simulink model "twip_control"  (R2015a)
settings: Solver=ode45  StartTime=0.0  StopTime=10  RelTol=1e-3
values from neighbouring files (symbols this model uses):
  s1 = 0.15    [Fuzzy_Balance_Controller_Mamdani.m]    (also in twip_sys.m = 1)
  s1_y = 0.5    [Fuzzy_Yaw_Controller_Mamdani.m]
  s2 = 0.4    [Fuzzy_Balance_Controller_Mamdani.m]    (also in twip_sys.m = 1)
  s2_y = 0.5    [Fuzzy_Yaw_Controller_Mamdani.m]
libraries: simulink x3, fuzblock x2
settings Model: Creator=elew  LastModifiedBy=ignacio
settings OptimizationCC: BlockReduction=off  OptimizeBlockIOStorage=off  BufferReuse=off  GlobalBufferReuse=off  ExpressionFolding=off  LocalBlockOutputs=off

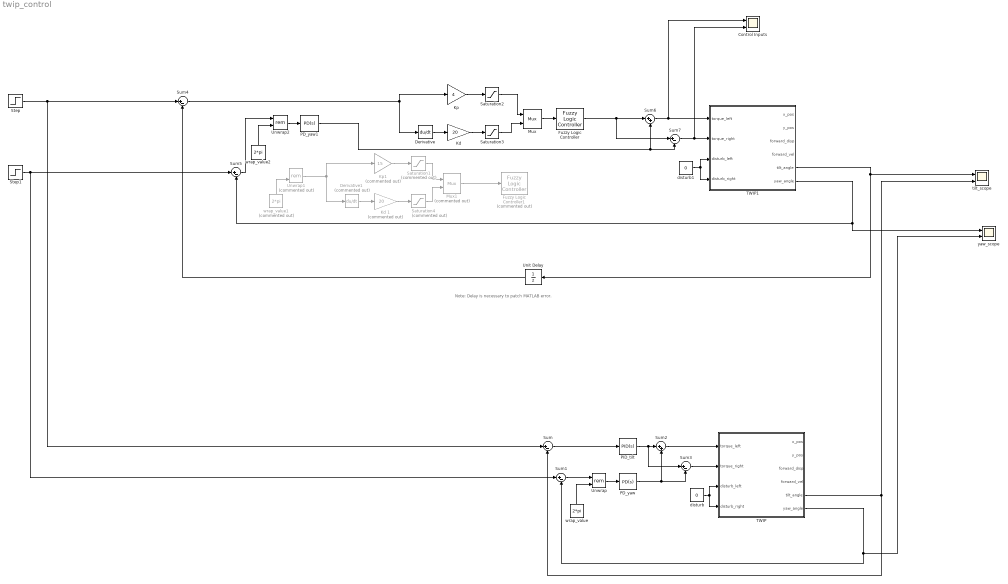
== system twip_control ==
  note: Note: Delay is necessary to patch MATLAB error.
  Control Inputs : Scope  NumInputPorts=2
      settings: YMin=-2~-2  YMax=1.5~1.5  SaveName=ScopeData2
  Derivative : Derivative
  Derivative1 : Derivative  Commented=on
  Fuzzy Logic Controller : fuzblock/Fuzzy Logic  Controller  fis='Bal.fis'
  Fuzzy Logic Controller1 : fuzblock/Fuzzy Logic  Controller  Commented=on  fis='Yaw.fis'
  "Kd " : Gain  Gain=20
  Kd 1 : Gain  Commented=on  Gain=20
  Kp : Gain  Gain=4
  Kp1 : Gain  Commented=on  Gain=15
  Mux : Mux  Inputs=2
      settings: DisplayOption=signals
  Mux1 : Mux  Commented=on  Inputs=2
      settings: DisplayOption=signals
  PD_yaw : simulink/Continuous/PID Controller  Controller=PD  TimeDomain=Continuous-time  SampleTime=-1  IntegratorMethod=Forward Euler  FilterMethod=Forward Euler  Form=Parallel  UseFilter=on  ControllerParametersSource=internal  P=25  I=100  D=1  N=100  InitialConditionSource=internal  InitialConditionForIntegrator=0  InitialConditionForFilter=0  ExternalReset=none  LimitOutput=off  UpperSaturationLimit=inf  LowerSaturationLimit=-inf  LinearizeAsGain=on  AntiWindupMode=none  Kb=1  TrackingMode=off  Kt=1  PParamMin=[]  PParamMax=[]  IParamMin=[]  IParamMax=[]  DParamMin=[]  DParamMax=[]  NParamMin=[]  NParamMax=[]  KbParamMin=[]  KbParamMax=[]  KtParamMin=[]  KtParamMax=[]  POutMin=[]  POutMax=[]  IOutMin=[]  IOutMax=[]  DOutMin=[]  DOutMax=[]  NOutMin=[]  NOutMax=[]  KbOutMin=[]  KbOutMax=[]  KtOutMin=[]  KtOutMax=[]  IntegratorOutMin=[]  IntegratorOutMax=[]  FilterOutMin=[]  FilterOutMax=[]  SumOutMin=[]  SumOutMax=[]  SumI1OutMin=[]  SumI1OutMax=[]  SumI2OutMin=[]  SumI2OutMax=[]  SumI3OutMin=[]  SumI3OutMax=[]  SumDOutMin=[]  SumDOutMax=[]  SaturationOutMin=[]  SaturationOutMax=[]  IntegratorContinuousStateAttributes=''  IntegratorStateMustResolveToSignalObject=off  IntegratorRTWStateStorageClass=Auto  FilterContinuousStateAttributes=''  FilterStateMustResolveToSignalObject=off  FilterRTWStateStorageClass=Auto  DifferentiatorICPrevScaledInput=0  DifferentiatorOutMin=[]  DifferentiatorOutMax=[]
  PD_yaw1 : simulink/Continuous/PID Controller  Controller=PD  TimeDomain=Continuous-time  SampleTime=-1  IntegratorMethod=Forward Euler  FilterMethod=Forward Euler  Form=Parallel  UseFilter=on  ControllerParametersSource=internal  P=25  I=100  D=1  N=100  InitialConditionSource=internal  InitialConditionForIntegrator=0  InitialConditionForFilter=0  ExternalReset=none  LimitOutput=off  UpperSaturationLimit=inf  LowerSaturationLimit=-inf  LinearizeAsGain=on  AntiWindupMode=none  Kb=1  TrackingMode=off  Kt=1  PParamMin=[]  PParamMax=[]  IParamMin=[]  IParamMax=[]  DParamMin=[]  DParamMax=[]  NParamMin=[]  NParamMax=[]  KbParamMin=[]  KbParamMax=[]  KtParamMin=[]  KtParamMax=[]  POutMin=[]  POutMax=[]  IOutMin=[]  IOutMax=[]  DOutMin=[]  DOutMax=[]  NOutMin=[]  NOutMax=[]  KbOutMin=[]  KbOutMax=[]  KtOutMin=[]  KtOutMax=[]  IntegratorOutMin=[]  IntegratorOutMax=[]  FilterOutMin=[]  FilterOutMax=[]  SumOutMin=[]  SumOutMax=[]  SumI1OutMin=[]  SumI1OutMax=[]  SumI2OutMin=[]  SumI2OutMax=[]  SumI3OutMin=[]  SumI3OutMax=[]  SumDOutMin=[]  SumDOutMax=[]  SaturationOutMin=[]  SaturationOutMax=[]  IntegratorContinuousStateAttributes=''  IntegratorStateMustResolveToSignalObject=off  IntegratorRTWStateStorageClass=Auto  FilterContinuousStateAttributes=''  FilterStateMustResolveToSignalObject=off  FilterRTWStateStorageClass=Auto  DifferentiatorICPrevScaledInput=0  DifferentiatorOutMin=[]  DifferentiatorOutMax=[]
  PID_tilt : simulink/Continuous/PID Controller  Controller=PID  TimeDomain=Continuous-time  SampleTime=-1  IntegratorMethod=Forward Euler  FilterMethod=Forward Euler  Form=Parallel  UseFilter=on  ControllerParametersSource=internal  P=50  I=100  D=2  N=100  InitialConditionSource=internal  InitialConditionForIntegrator=0  InitialConditionForFilter=0  ExternalReset=none  LimitOutput=off  UpperSaturationLimit=inf  LowerSaturationLimit=-inf  LinearizeAsGain=on  AntiWindupMode=none  Kb=1  TrackingMode=off  Kt=1  PParamMin=[]  PParamMax=[]  IParamMin=[]  IParamMax=[]  DParamMin=[]  DParamMax=[]  NParamMin=[]  NParamMax=[]  KbParamMin=[]  KbParamMax=[]  KtParamMin=[]  KtParamMax=[]  POutMin=[]  POutMax=[]  IOutMin=[]  IOutMax=[]  DOutMin=[]  DOutMax=[]  NOutMin=[]  NOutMax=[]  KbOutMin=[]  KbOutMax=[]  KtOutMin=[]  KtOutMax=[]  IntegratorOutMin=[]  IntegratorOutMax=[]  FilterOutMin=[]  FilterOutMax=[]  SumOutMin=[]  SumOutMax=[]  SumI1OutMin=[]  SumI1OutMax=[]  SumI2OutMin=[]  SumI2OutMax=[]  SumI3OutMin=[]  SumI3OutMax=[]  SumDOutMin=[]  SumDOutMax=[]  SaturationOutMin=[]  SaturationOutMax=[]  IntegratorContinuousStateAttributes=''  IntegratorStateMustResolveToSignalObject=off  IntegratorRTWStateStorageClass=Auto  FilterContinuousStateAttributes=''  FilterStateMustResolveToSignalObject=off  FilterRTWStateStorageClass=Auto  DifferentiatorICPrevScaledInput=0  DifferentiatorOutMin=[]  DifferentiatorOutMax=[]
  Saturation1 : Saturate  Commented=on  UpperLimit=1*s1_y  LowerLimit=-1*s1_y  ZeroCross=off
  Saturation2 : Saturate  UpperLimit=6*s1  LowerLimit=-6*s1  ZeroCross=off
  Saturation3 : Saturate  UpperLimit=2*s2  LowerLimit=-2*s2  ZeroCross=off
  Saturation4 : Saturate  Commented=on  UpperLimit=1*s2_y  LowerLimit=-1*s2_y  ZeroCross=off
  Step : Step  After=-0.3  SampleTime=0
  Step1 : Step  After=0.1  SampleTime=0
  Sum{,1,3..5,7} (6 alike) : Sum  Inputs=|+-
  Sum2 : Sum  Inputs=|++
  Sum6 : Sum  Inputs=|++
  TWIP : Subsystem
      mask Display:
      | image('twip_mask.png')
      | port_label('input', 1, 'torque_l')
      | port_label('input', 2, 'torque_r')
      | port_label('input', 3, 'disturb_l')
      | port_label('input', 4, 'disturb_r')
      | 
      | 
      | port_label('output', 1, 'x_pos')
      | port_label('output', 2, 'y_pos')
      | port_label('output', 3, 'disp')
      | port_label('output', 4, 'vel')
      | port_label('output', 5, 'tilt')
      | port_label('output', 6, 'yaw')
  TWIP1 : Subsystem
      mask Display:
      | image('twip_mask.png')
      | port_label('input', 1, 'torque_l')
      | port_label('input', 2, 'torque_r')
      | port_label('input', 3, 'disturb_l')
      | port_label('input', 4, 'disturb_r')
      | 
      | 
      | port_label('output', 1, 'x_pos')
      | port_label('output', 2, 'y_pos')
      | port_label('output', 3, 'disp')
      | port_label('output', 4, 'vel')
      | port_label('output', 5, 'tilt')
      | port_label('output', 6, 'yaw')
  Unit Delay : UnitDelay  SampleTime=0.01
  Unwrap : Math  Operator=rem  SaturateOnIntegerOverflow=on
  Unwrap1 : Math  Commented=on  Operator=rem  SaturateOnIntegerOverflow=on
  Unwrap2 : Math  Operator=rem  SaturateOnIntegerOverflow=on
  disturb : Constant  Value=0
  disturb1 : Constant  Value=0
  "tilt_scope " : Scope  NumInputPorts=2
      settings: ShowLegends=on  TimeRange=2.2890625  YMin=-0.303~-0.301  YMax=-0.29775~-0.2915  SaveName=ScopeData4
  wrap_value : Constant  Value=2*pi
  wrap_value1 : Constant  Commented=on  Value=2*pi
  wrap_value2 : Constant  Value=2*pi
  yaw_scope : Scope  NumInputPorts=2
      settings: YMin=0.1~0.1  YMax=0.1~0.1  SaveName=ScopeData5
  wires:
  TWIP/5(tilt_angle) -> Sum/2, "tilt_scope "/2
  Sum/1 -> PID_tilt/1
  disturb/1 -> TWIP/4(disturb_right), TWIP/3(disturb_left)
  TWIP/6(yaw_angle) -> yaw_scope/2, Sum1/2
  Sum1/1 -> Unwrap/1
  Sum2/1 -> TWIP/1(torque_left)
  Sum3/1 -> TWIP/2(torque_right)
  Unwrap/1 -> PD_yaw/1
  wrap_value/1 -> Unwrap/2
  disturb1/1 -> TWIP1/4(disturb_right), TWIP1/3(disturb_left)
  Sum7/1 -> Control Inputs/2, TWIP1/2(torque_right)
  wrap_value1/1 -> Unwrap1/2
  TWIP1/5(tilt_angle) -> Unit Delay/1, "tilt_scope "/1
  Derivative/1 -> "Kd "/1
  Unit Delay/1 -> Sum4/2
  Sum4/1 -> Derivative/1, Kp/1
  Mux/1 -> Fuzzy Logic Controller/1
  Kp/1 -> Saturation2/1
  "Kd "/1 -> Saturation3/1
  Saturation2/1 -> Mux/1
  Saturation3/1 -> Mux/2
  Derivative1/1 -> Kd 1/1
  Unwrap1/1 -> Kp1/1, Derivative1/1
  Mux1/1 -> Fuzzy Logic Controller1/1
  Kp1/1 -> Saturation1/1
  Kd 1/1 -> Saturation4/1
  Saturation1/1 -> Mux1/1
  Saturation4/1 -> Mux1/2
  PID_tilt/1 -> Sum3/1, Sum2/1
  Step/1 -> Sum/1, Sum4/1
  Step1/1 -> Sum5/1, Sum1/1
  Sum5/1 -> Unwrap2/1
  Unwrap2/1 -> PD_yaw1/1
  wrap_value2/1 -> Unwrap2/2
  Fuzzy Logic Controller/1 -> Sum7/1, Sum6/1
  PD_yaw/1 -> Sum3/2, Sum2/2
  Sum6/1 -> Control Inputs/1, TWIP1/1(torque_left)
  PD_yaw1/1 -> Sum7/2, Sum6/2
  TWIP1/6(yaw_angle) -> Sum5/2, yaw_scope/1

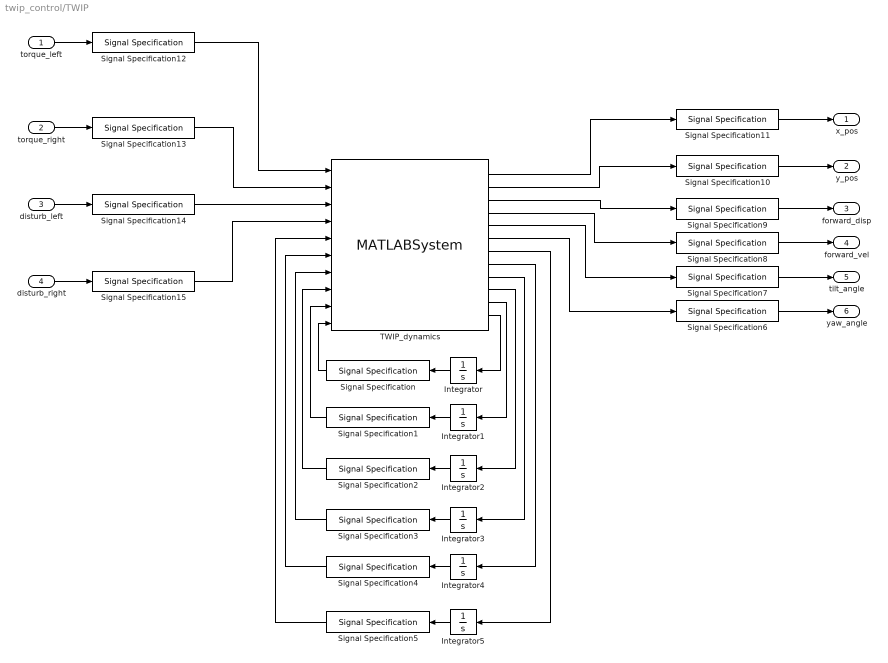
== system twip_control/TWIP ==
  torque_left : Inport
  torque_right : Inport  Port=2
  disturb_left : Inport  Port=3
  disturb_right : Inport  Port=4
  Integrator{,1..4} (5 alike) : Integrator
  Integrator5 : Integrator  InitialCondition=0.3
  Signal Specification{,1..15} (16 alike) : SignalSpecification  Dimensions=[1]
  TWIP_dynamics : MATLABSystem  System=twip_sys  M=[0.5]  Mw=[0.8]  mm=[0.5]  Iw=[0.02]  Ip=[0.06]  Imm=[0.08]  r=[0.2]  l=[0.15]  d=[0.6]  SimulateUsing=Interpreted execution
      mask Type: twip_sys
      mask Display:
      | disp('twip_sys');
      | port_label('input',1,'tl');
      | port_label('input',2,'tr');
      | port_label('input',3,'dl');
      | port_label('input',4,'dr');
      | port_label('input',5,'y1');
      | port_label('input',6,'y2');
      | port_label('input',7,'y3');
      | port_label('input',8,'y4');
      | port_label('input',9,'y5');
      | port_label('input',10,'y6');
      | port_label('output',1,'x');
      | port_label('output',2,'y');
      | port_label('output',3,'xp');
      | port_label('output',4,'v');
      | port_label('output',5,'alpha');
      | port_label('output',6,'theta');
      | port_label('output',7,'yd1');
      | port_label('output',8,'yd2');
      | port_label('output',9,'yd3');
      | port_label('output',10,'yd4');
      | port_label('output',11,'yd5');
      | port_label('output',12,'yd6');
  x_pos : Outport
  y_pos : Outport  Port=2
  forward_disp : Outport  Port=3
  forward_vel : Outport  Port=4
  tilt_angle : Outport  Port=5
  yaw_angle : Outport  Port=6
  wires:
  torque_right/1 -> Signal Specification13/1
  torque_left/1 -> Signal Specification12/1
  disturb_right/1 -> Signal Specification15/1
  disturb_left/1 -> Signal Specification14/1
  TWIP_dynamics/1 -> Signal Specification11/1
  TWIP_dynamics/2 -> Signal Specification10/1
  TWIP_dynamics/3 -> Signal Specification9/1
  TWIP_dynamics/4 -> Signal Specification8/1
  TWIP_dynamics/5 -> Signal Specification7/1
  TWIP_dynamics/6 -> Signal Specification6/1
  TWIP_dynamics/12 -> Integrator/1
  Integrator/1 -> Signal Specification/1
  Integrator1/1 -> Signal Specification1/1
  Integrator2/1 -> Signal Specification2/1
  Integrator3/1 -> Signal Specification3/1
  Integrator4/1 -> Signal Specification4/1
  Integrator5/1 -> Signal Specification5/1
  TWIP_dynamics/11 -> Integrator1/1
  TWIP_dynamics/10 -> Integrator2/1
  TWIP_dynamics/9 -> Integrator3/1
  TWIP_dynamics/8 -> Integrator4/1
  TWIP_dynamics/7 -> Integrator5/1
  Signal Specification/1 -> TWIP_dynamics/10
  Signal Specification1/1 -> TWIP_dynamics/9
  Signal Specification2/1 -> TWIP_dynamics/8
  Signal Specification3/1 -> TWIP_dynamics/7
  Signal Specification4/1 -> TWIP_dynamics/6
  Signal Specification5/1 -> TWIP_dynamics/5
  Signal Specification6/1 -> yaw_angle/1
  Signal Specification7/1 -> tilt_angle/1
  Signal Specification8/1 -> forward_vel/1
  Signal Specification9/1 -> forward_disp/1
  Signal Specification10/1 -> y_pos/1
  Signal Specification11/1 -> x_pos/1
  Signal Specification12/1 -> TWIP_dynamics/1
  Signal Specification13/1 -> TWIP_dynamics/2
  Signal Specification14/1 -> TWIP_dynamics/3
  Signal Specification15/1 -> TWIP_dynamics/4

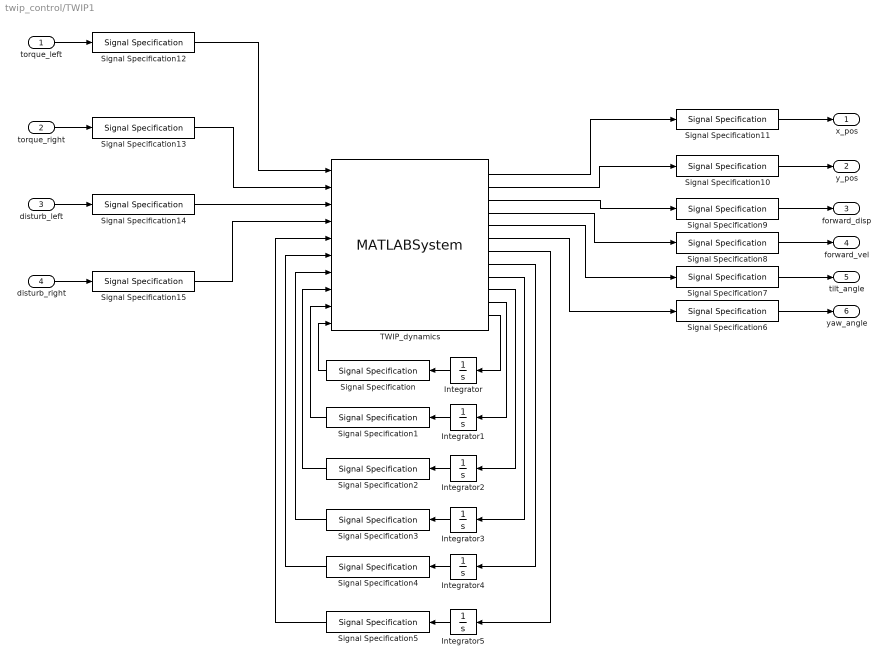
== system twip_control/TWIP1 ==
  torque_left : Inport
  torque_right : Inport  Port=2
  disturb_left : Inport  Port=3
  disturb_right : Inport  Port=4
  Integrator{,1..4} (5 alike) : Integrator
  Integrator5 : Integrator  InitialCondition=0.3
  Signal Specification{,1..15} (16 alike) : SignalSpecification  Dimensions=[1]
  TWIP_dynamics : MATLABSystem  System=twip_sys  M=[0.5]  Mw=[0.8]  mm=[0.5]  Iw=[0.02]  Ip=[0.06]  Imm=[0.08]  r=[0.2]  l=[0.15]  d=[0.6]  SimulateUsing=Interpreted execution
      mask Type: twip_sys
      mask Display:
      | disp('twip_sys');
      | port_label('input',1,'tl');
      | port_label('input',2,'tr');
      | port_label('input',3,'dl');
      | port_label('input',4,'dr');
      | port_label('input',5,'y1');
      | port_label('input',6,'y2');
      | port_label('input',7,'y3');
      | port_label('input',8,'y4');
      | port_label('input',9,'y5');
      | port_label('input',10,'y6');
      | port_label('output',1,'x');
      | port_label('output',2,'y');
      | port_label('output',3,'xp');
      | port_label('output',4,'v');
      | port_label('output',5,'alpha');
      | port_label('output',6,'theta');
      | port_label('output',7,'yd1');
      | port_label('output',8,'yd2');
      | port_label('output',9,'yd3');
      | port_label('output',10,'yd4');
      | port_label('output',11,'yd5');
      | port_label('output',12,'yd6');
  x_pos : Outport
  y_pos : Outport  Port=2
  forward_disp : Outport  Port=3
  forward_vel : Outport  Port=4
  tilt_angle : Outport  Port=5
  yaw_angle : Outport  Port=6
  wires:
  torque_right/1 -> Signal Specification13/1
  torque_left/1 -> Signal Specification12/1
  disturb_right/1 -> Signal Specification15/1
  disturb_left/1 -> Signal Specification14/1
  TWIP_dynamics/1 -> Signal Specification11/1
  TWIP_dynamics/2 -> Signal Specification10/1
  TWIP_dynamics/3 -> Signal Specification9/1
  TWIP_dynamics/4 -> Signal Specification8/1
  TWIP_dynamics/5 -> Signal Specification7/1
  TWIP_dynamics/6 -> Signal Specification6/1
  TWIP_dynamics/12 -> Integrator/1
  Integrator/1 -> Signal Specification/1
  Integrator1/1 -> Signal Specification1/1
  Integrator2/1 -> Signal Specification2/1
  Integrator3/1 -> Signal Specification3/1
  Integrator4/1 -> Signal Specification4/1
  Integrator5/1 -> Signal Specification5/1
  TWIP_dynamics/11 -> Integrator1/1
  TWIP_dynamics/10 -> Integrator2/1
  TWIP_dynamics/9 -> Integrator3/1
  TWIP_dynamics/8 -> Integrator4/1
  TWIP_dynamics/7 -> Integrator5/1
  Signal Specification/1 -> TWIP_dynamics/10
  Signal Specification1/1 -> TWIP_dynamics/9
  Signal Specification2/1 -> TWIP_dynamics/8
  Signal Specification3/1 -> TWIP_dynamics/7
  Signal Specification4/1 -> TWIP_dynamics/6
  Signal Specification5/1 -> TWIP_dynamics/5
  Signal Specification6/1 -> yaw_angle/1
  Signal Specification7/1 -> tilt_angle/1
  Signal Specification8/1 -> forward_vel/1
  Signal Specification9/1 -> forward_disp/1
  Signal Specification10/1 -> y_pos/1
  Signal Specification11/1 -> x_pos/1
  Signal Specification12/1 -> TWIP_dynamics/1
  Signal Specification13/1 -> TWIP_dynamics/2
  Signal Specification14/1 -> TWIP_dynamics/3
  Signal Specification15/1 -> TWIP_dynamics/4
